simulink model "UnifiedPowerFlowController"  (R2024a)
settings: Solver=FixedStepDiscrete  StartTime=0.0  StopTime=0.8  FixedStep=Ts  RelTol=1e-3
PreLoadFcn:
  | Ts=1/512/60;
undefined symbols (not defined in the file or in its folder): DiscIntNeverNeededParam
libraries: spsabctodq0Lib x10, spsMeanVariableFrequencyLib x10, spsThreeLevelBridgeLib x8, spsVoltageMeasurementLib x8, spsZigzagPhaseShiftingTransformerLib x8, spsCurrentMeasurementLib x6, spsSecondOrderFilterLib x5, spsThreePhaseVIMeasurementLib x4, spsSeriesRLCBranchLib x4, spsDistributedParametersLineLib x3, spsPowerPositiveSequenceLib x3, spsThreePhaseSourceLib x2
(part 5 of 7)

== system UnifiedPowerFlowController/UPFC Controller/SE Control (SSSC)/Firing Pulses Generator/Bridge 1Y /Phase B ==
  note: <--Sigma-->
  note: |
      | |
      | |
  note: |
      | |
      | |
  note: Q4
  note: Q3
  note: Q2
  note: Q1
  note: ******************************************
  note: ********************************************
  note: ******************
  note: ******************
  note: 360
  note: 180
  note: 0
  note: I--------------------------------I-----------------------------I--
  note: Normal 180deg
      | Operation
  note: Normal 180deg
      | Operation
  note: Normal 180deg
      | Operation
  note: Pulses timing
      | ===========
  note: |
      | |
      | |
      | |
      | |
      | |
      | |
      | |
      | |
      | |
      | |
  note: |
      | |
      | |
      | |
      | |
      | |
      | |
      | |
      | |
      | |
      | |
  note: |
      | |
      | |
      | |
      | |
      | |
      | |
      | |
      | |
      | |
      | |
  note: Q1,Q2,Q3,Q4
  note: Q2,Q3
  note: Q4,Q1
  note: + Vdc -------------------------------
  note: - Vdc -------------------------------
  note: N -------
  note: |
      | |
      | |
      | |
      | |
      | |
      | |
      | |
      | |
      | |
      | |
  note: ---------- A
  note: --------[D-NN]---------
  note: --------[D_NP]---------
  note: |
      | |
      | [G4]
      | |
      | |
      | |
  note: |
      | |
      | [Q3]
      | |
      | |
  note: |
      | |
      | [Q2]
      | |
      | |
  note: |
      | |
      | |
      | [Q1]
      | |
      | |
  wt : Inport  PortDimensions=1
  sigma : Inport  Port=2  PortDimensions=1
  D_Alpha : Inport  Port=3  PortDimensions=1
  Constant1 : Constant  Value=[0 -pi]
  Constant2 : Constant  Value=2*pi
  Constant3 : Constant  Value=0
  Constant8 : Constant  Value=pi
  Constant9 : Constant  Value=pi
  Deg->Rad2 : Gain  Gain=0.5  SaturateOnIntegerOverflow=on  OutDataTypeStr=Inherit: Same as input  ParamDataTypeStr=Inherit: Same as input
  Deg->Rad3 : Gain  Gain=-1  SaturateOnIntegerOverflow=on  OutDataTypeStr=Inherit: Same as input  ParamDataTypeStr=Inherit: Same as input
  Gain3 : Gain  Gain=2  SaturateOnIntegerOverflow=on  OutDataTypeStr=Inherit: Same as input  ParamDataTypeStr=Inherit: Same as input
  Logical Operator : Logic
  Logical Operator2 : Logic  Operator=NOT
  Math Function : Math  Operator=mod  SignedPower=on
  Mux3 : Mux  Inputs=[2 2]
  Mux4 : Mux  Inputs=2
  Relational Operator : RelationalOperator
  Relational Operator1 : RelationalOperator  Operator=<
  Selector3 : Selector  InputPortWidth=4  IndexOptions=Index vector (dialog)  Indices=[4 1 2 3]  OutputSizes=1
  Sum{2,4..6} (4 alike) : Sum  InputSameDT=on  SaturateOnIntegerOverflow=on  OutDataTypeStr=Inherit: Same as first input
  Sum3 : Sum  Inputs=+-  InputSameDT=on  SaturateOnIntegerOverflow=on  OutDataTypeStr=Inherit: Same as first input
  Pulses : Outport  VectorParamsAs1DForOutWhenUnconnected=off
  wires:
  Constant2/1 -> Math Function/2
  Sum5/1 -> Sum2/1  "theta"
  wt/1 -> Sum5/1  "wt"
  D_Alpha/1 -> Mux4/1, Deg->Rad3/1
  Deg->Rad3/1 -> Mux4/2
  Mux4/1 -> Sum5/2
  Math Function/1 -> Relational Operator/1, Relational Operator1/1
  Gain3/1 -> Sum6/1
  Selector3/1 -> Pulses/1
  Mux3/1 -> Selector3/1
  Logical Operator2/1 -> Mux3/2
  Logical Operator/1 -> Mux3/1, Logical Operator2/1
  Sum4/1 -> Math Function/1
  Sum2/1 -> Sum4/2
  Sum6/1 -> Relational Operator1/2
  Constant8/1 -> Sum6/2
  Deg->Rad2/1 -> Gain3/1, Sum4/1  "Beta"
  Sum3/1 -> Deg->Rad2/1
  sigma/1 -> Sum3/2
  Constant9/1 -> Sum3/1
  Relational Operator1/1 -> Logical Operator/2
  Relational Operator/1 -> Logical Operator/1
  Constant3/1 -> Relational Operator/2
  Constant1/1 -> Sum2/2

== system UnifiedPowerFlowController/UPFC Controller/SE Control (SSSC)/Firing Pulses Generator/Bridge 1Y /Phase C ==
  note: |
      | |
      | |
      | [Q1]
      | |
      | |
  note: |
      | |
      | [Q2]
      | |
      | |
  note: |
      | |
      | [Q3]
      | |
      | |
  note: |
      | |
      | [G4]
      | |
      | |
      | |
  note: --------[D_NP]---------
  note: --------[D-NN]---------
  note: ---------- A
  note: |
      | |
      | |
      | |
      | |
      | |
      | |
      | |
      | |
      | |
      | |
  note: N -------
  note: - Vdc -------------------------------
  note: + Vdc -------------------------------
  note: Q4,Q1
  note: Q2,Q3
  note: Q1,Q2,Q3,Q4
  note: |
      | |
      | |
      | |
      | |
      | |
      | |
      | |
      | |
      | |
      | |
  note: |
      | |
      | |
      | |
      | |
      | |
      | |
      | |
      | |
      | |
      | |
  note: |
      | |
      | |
      | |
      | |
      | |
      | |
      | |
      | |
      | |
      | |
  note: Pulses timing
      | ===========
  note: Normal 180deg
      | Operation
  note: Normal 180deg
      | Operation
  note: Normal 180deg
      | Operation
  note: I--------------------------------I-----------------------------I--
  note: 0
  note: 180
  note: 360
  note: ******************
  note: ******************
  note: ********************************************
  note: ******************************************
  note: Q1
  note: Q2
  note: Q3
  note: Q4
  note: |
      | |
      | |
  note: |
      | |
      | |
  note: <--Sigma-->
  wt : Inport  PortDimensions=1
  sigma : Inport  Port=2  PortDimensions=1
  D_Alpha : Inport  Port=3  PortDimensions=1
  Constant1 : Constant  Value=[0 -pi]
  Constant2 : Constant  Value=2*pi
  Constant3 : Constant  Value=0
  Constant8 : Constant  Value=pi
  Constant9 : Constant  Value=pi
  Deg->Rad2 : Gain  Gain=0.5  SaturateOnIntegerOverflow=on  OutDataTypeStr=Inherit: Same as input  ParamDataTypeStr=Inherit: Same as input
  Deg->Rad3 : Gain  Gain=-1  SaturateOnIntegerOverflow=on  OutDataTypeStr=Inherit: Same as input  ParamDataTypeStr=Inherit: Same as input
  Gain3 : Gain  Gain=2  SaturateOnIntegerOverflow=on  OutDataTypeStr=Inherit: Same as input  ParamDataTypeStr=Inherit: Same as input
  Logical Operator : Logic
  Logical Operator2 : Logic  Operator=NOT
  Math Function : Math  Operator=mod  SignedPower=on
  Mux3 : Mux  Inputs=[2 2]
  Mux4 : Mux  Inputs=2
  Relational Operator : RelationalOperator
  Relational Operator1 : RelationalOperator  Operator=<
  Selector3 : Selector  InputPortWidth=4  IndexOptions=Index vector (dialog)  Indices=[4 1 2 3]  OutputSizes=1
  Sum{2,4..6} (4 alike) : Sum  InputSameDT=on  SaturateOnIntegerOverflow=on  OutDataTypeStr=Inherit: Same as first input
  Sum3 : Sum  Inputs=+-  InputSameDT=on  SaturateOnIntegerOverflow=on  OutDataTypeStr=Inherit: Same as first input
  Pulses : Outport  VectorParamsAs1DForOutWhenUnconnected=off
  wires:
  Constant1/1 -> Sum2/2
  Constant3/1 -> Relational Operator/2
  Relational Operator/1 -> Logical Operator/1
  Relational Operator1/1 -> Logical Operator/2
  Constant9/1 -> Sum3/1
  sigma/1 -> Sum3/2
  Sum3/1 -> Deg->Rad2/1
  Deg->Rad2/1 -> Sum4/1, Gain3/1  "Beta"
  Constant8/1 -> Sum6/2
  Sum6/1 -> Relational Operator1/2
  Sum2/1 -> Sum4/2
  Sum4/1 -> Math Function/1
  Logical Operator/1 -> Logical Operator2/1, Mux3/1
  Logical Operator2/1 -> Mux3/2
  Mux3/1 -> Selector3/1
  Selector3/1 -> Pulses/1
  Gain3/1 -> Sum6/1
  Math Function/1 -> Relational Operator1/1, Relational Operator/1
  Mux4/1 -> Sum5/2
  Deg->Rad3/1 -> Mux4/2
  D_Alpha/1 -> Deg->Rad3/1, Mux4/1
  wt/1 -> Sum5/1  "wt"
  Sum5/1 -> Sum2/1  "theta"
  Constant2/1 -> Math Function/2

== system UnifiedPowerFlowController/UPFC Controller/SE Control (SSSC)/Firing Pulses Generator/Bridge 2D/Phase A ==
  note: <--Sigma-->
  note: |
      | |
      | |
  note: |
      | |
      | |
  note: Q4
  note: Q3
  note: Q2
  note: Q1
  note: ******************************************
  note: ********************************************
  note: ******************
  note: ******************
  note: 360
  note: 180
  note: 0
  note: I--------------------------------I-----------------------------I--
  note: Normal 180deg
      | Operation
  note: Normal 180deg
      | Operation
  note: Normal 180deg
      | Operation
  note: Pulses timing
      | ===========
  note: |
      | |
      | |
      | |
      | |
      | |
      | |
      | |
      | |
      | |
      | |
  note: |
      | |
      | |
      | |
      | |
      | |
      | |
      | |
      | |
      | |
      | |
  note: |
      | |
      | |
      | |
      | |
      | |
      | |
      | |
      | |
      | |
      | |
  note: Q1,Q2,Q3,Q4
  note: Q2,Q3
  note: Q4,Q1
  note: + Vdc -------------------------------
  note: - Vdc -------------------------------
  note: N -------
  note: |
      | |
      | |
      | |
      | |
      | |
      | |
      | |
      | |
      | |
      | |
  note: ---------- A
  note: --------[D-NN]---------
  note: --------[D_NP]---------
  note: |
      | |
      | [G4]
      | |
      | |
      | |
  note: |
      | |
      | [Q3]
      | |
      | |
  note: |
      | |
      | [Q2]
      | |
      | |
  note: |
      | |
      | |
      | [Q1]
      | |
      | |
  wt : Inport  PortDimensions=1
  sigma : Inport  Port=2  PortDimensions=1
  D_Alpha : Inport  Port=3  PortDimensions=1
  Constant1 : Constant  Value=[0 -pi]
  Constant2 : Constant  Value=2*pi
  Constant3 : Constant  Value=0
  Constant8 : Constant  Value=pi
  Constant9 : Constant  Value=pi
  Deg->Rad2 : Gain  Gain=0.5  SaturateOnIntegerOverflow=on  OutDataTypeStr=Inherit: Same as input  ParamDataTypeStr=Inherit: Same as input
  Deg->Rad3 : Gain  Gain=-1  SaturateOnIntegerOverflow=on  OutDataTypeStr=Inherit: Same as input  ParamDataTypeStr=Inherit: Same as input
  Gain3 : Gain  Gain=2  SaturateOnIntegerOverflow=on  OutDataTypeStr=Inherit: Same as input  ParamDataTypeStr=Inherit: Same as input
  Logical Operator : Logic
  Logical Operator2 : Logic  Operator=NOT
  Math Function : Math  Operator=mod  SignedPower=on
  Mux3 : Mux  Inputs=[2 2]
  Mux4 : Mux  Inputs=2
  Relational Operator : RelationalOperator
  Relational Operator1 : RelationalOperator  Operator=<
  Selector3 : Selector  InputPortWidth=4  IndexOptions=Index vector (dialog)  Indices=[4 1 2 3]  OutputSizes=1
  Sum{2,4..6} (4 alike) : Sum  InputSameDT=on  SaturateOnIntegerOverflow=on  OutDataTypeStr=Inherit: Same as first input
  Sum3 : Sum  Inputs=+-  InputSameDT=on  SaturateOnIntegerOverflow=on  OutDataTypeStr=Inherit: Same as first input
  Pulses : Outport  VectorParamsAs1DForOutWhenUnconnected=off
  wires:
  Constant2/1 -> Math Function/2
  Sum5/1 -> Sum2/1  "theta"
  wt/1 -> Sum5/1  "wt"
  D_Alpha/1 -> Mux4/1, Deg->Rad3/1
  Deg->Rad3/1 -> Mux4/2
  Mux4/1 -> Sum5/2
  Math Function/1 -> Relational Operator/1, Relational Operator1/1
  Gain3/1 -> Sum6/1
  Selector3/1 -> Pulses/1
  Mux3/1 -> Selector3/1
  Logical Operator2/1 -> Mux3/2
  Logical Operator/1 -> Mux3/1, Logical Operator2/1
  Sum4/1 -> Math Function/1
  Sum2/1 -> Sum4/2
  Sum6/1 -> Relational Operator1/2
  Constant8/1 -> Sum6/2
  Deg->Rad2/1 -> Gain3/1, Sum4/1  "Beta"
  Sum3/1 -> Deg->Rad2/1
  sigma/1 -> Sum3/2
  Constant9/1 -> Sum3/1
  Relational Operator1/1 -> Logical Operator/2
  Relational Operator/1 -> Logical Operator/1
  Constant3/1 -> Relational Operator/2
  Constant1/1 -> Sum2/2

== system UnifiedPowerFlowController/UPFC Controller/SE Control (SSSC)/Firing Pulses Generator/Bridge 2D/Phase B ==
  note: |
      | |
      | |
      | [Q1]
      | |
      | |
  note: |
      | |
      | [Q2]
      | |
      | |
  note: |
      | |
      | [Q3]
      | |
      | |
  note: |
      | |
      | [G4]
      | |
      | |
      | |
  note: --------[D_NP]---------
  note: --------[D-NN]---------
  note: ---------- A
  note: |
      | |
      | |
      | |
      | |
      | |
      | |
      | |
      | |
      | |
      | |
  note: N -------
  note: - Vdc -------------------------------
  note: + Vdc -------------------------------
  note: Q4,Q1
  note: Q2,Q3
  note: Q1,Q2,Q3,Q4
  note: |
      | |
      | |
      | |
      | |
      | |
      | |
      | |
      | |
      | |
      | |
  note: |
      | |
      | |
      | |
      | |
      | |
      | |
      | |
      | |
      | |
      | |
  note: |
      | |
      | |
      | |
      | |
      | |
      | |
      | |
      | |
      | |
      | |
  note: Pulses timing
      | ===========
  note: Normal 180deg
      | Operation
  note: Normal 180deg
      | Operation
  note: Normal 180deg
      | Operation
  note: I--------------------------------I-----------------------------I--
  note: 0
  note: 180
  note: 360
  note: ******************
  note: ******************
  note: ********************************************
  note: ******************************************
  note: Q1
  note: Q2
  note: Q3
  note: Q4
  note: |
      | |
      | |
  note: |
      | |
      | |
  note: <--Sigma-->
  wt : Inport  PortDimensions=1
  sigma : Inport  Port=2  PortDimensions=1
  D_Alpha : Inport  Port=3  PortDimensions=1
  Constant1 : Constant  Value=[0 -pi]
  Constant2 : Constant  Value=2*pi
  Constant3 : Constant  Value=0
  Constant8 : Constant  Value=pi
  Constant9 : Constant  Value=pi
  Deg->Rad2 : Gain  Gain=0.5  SaturateOnIntegerOverflow=on  OutDataTypeStr=Inherit: Same as input  ParamDataTypeStr=Inherit: Same as input
  Deg->Rad3 : Gain  Gain=-1  SaturateOnIntegerOverflow=on  OutDataTypeStr=Inherit: Same as input  ParamDataTypeStr=Inherit: Same as input
  Gain3 : Gain  Gain=2  SaturateOnIntegerOverflow=on  OutDataTypeStr=Inherit: Same as input  ParamDataTypeStr=Inherit: Same as input
  Logical Operator : Logic
  Logical Operator2 : Logic  Operator=NOT
  Math Function : Math  Operator=mod  SignedPower=on
  Mux3 : Mux  Inputs=[2 2]
  Mux4 : Mux  Inputs=2
  Relational Operator : RelationalOperator
  Relational Operator1 : RelationalOperator  Operator=<
  Selector3 : Selector  InputPortWidth=4  IndexOptions=Index vector (dialog)  Indices=[4 1 2 3]  OutputSizes=1
  Sum{2,4..6} (4 alike) : Sum  InputSameDT=on  SaturateOnIntegerOverflow=on  OutDataTypeStr=Inherit: Same as first input
  Sum3 : Sum  Inputs=+-  InputSameDT=on  SaturateOnIntegerOverflow=on  OutDataTypeStr=Inherit: Same as first input
  Pulses : Outport  VectorParamsAs1DForOutWhenUnconnected=off
  wires:
  Constant1/1 -> Sum2/2
  Constant3/1 -> Relational Operator/2
  Relational Operator/1 -> Logical Operator/1
  Relational Operator1/1 -> Logical Operator/2
  Constant9/1 -> Sum3/1
  sigma/1 -> Sum3/2
  Sum3/1 -> Deg->Rad2/1
  Deg->Rad2/1 -> Sum4/1, Gain3/1  "Beta"
  Constant8/1 -> Sum6/2
  Sum6/1 -> Relational Operator1/2
  Sum2/1 -> Sum4/2
  Sum4/1 -> Math Function/1
  Logical Operator/1 -> Logical Operator2/1, Mux3/1
  Logical Operator2/1 -> Mux3/2
  Mux3/1 -> Selector3/1
  Selector3/1 -> Pulses/1
  Gain3/1 -> Sum6/1
  Math Function/1 -> Relational Operator1/1, Relational Operator/1
  Mux4/1 -> Sum5/2
  Deg->Rad3/1 -> Mux4/2
  D_Alpha/1 -> Deg->Rad3/1, Mux4/1
  wt/1 -> Sum5/1  "wt"
  Sum5/1 -> Sum2/1  "theta"
  Constant2/1 -> Math Function/2

== system UnifiedPowerFlowController/UPFC Controller/SE Control (SSSC)/Firing Pulses Generator/Bridge 2D/Phase C ==
  note: <--Sigma-->
  note: |
      | |
      | |
  note: |
      | |
      | |
  note: Q4
  note: Q3
  note: Q2
  note: Q1
  note: ******************************************
  note: ********************************************
  note: ******************
  note: ******************
  note: 360
  note: 180
  note: 0
  note: I--------------------------------I-----------------------------I--
  note: Normal 180deg
      | Operation
  note: Normal 180deg
      | Operation
  note: Normal 180deg
      | Operation
  note: Pulses timing
      | ===========
  note: |
      | |
      | |
      | |
      | |
      | |
      | |
      | |
      | |
      | |
      | |
  note: |
      | |
      | |
      | |
      | |
      | |
      | |
      | |
      | |
      | |
      | |
  note: |
      | |
      | |
      | |
      | |
      | |
      | |
      | |
      | |
      | |
      | |
  note: Q1,Q2,Q3,Q4
  note: Q2,Q3
  note: Q4,Q1
  note: + Vdc -------------------------------
  note: - Vdc -------------------------------
  note: N -------
  note: |
      | |
      | |
      | |
      | |
      | |
      | |
      | |
      | |
      | |
      | |
  note: ---------- A
  note: --------[D-NN]---------
  note: --------[D_NP]---------
  note: |
      | |
      | [G4]
      | |
      | |
      | |
  note: |
      | |
      | [Q3]
      | |
      | |
  note: |
      | |
      | [Q2]
      | |
      | |
  note: |
      | |
      | |
      | [Q1]
      | |
      | |
  wt : Inport  PortDimensions=1
  sigma : Inport  Port=2  PortDimensions=1
  D_Alpha : Inport  Port=3  PortDimensions=1
  Constant1 : Constant  Value=[0 -pi]
  Constant2 : Constant  Value=2*pi
  Constant3 : Constant  Value=0
  Constant8 : Constant  Value=pi
  Constant9 : Constant  Value=pi
  Deg->Rad2 : Gain  Gain=0.5  SaturateOnIntegerOverflow=on  OutDataTypeStr=Inherit: Same as input  ParamDataTypeStr=Inherit: Same as input
  Deg->Rad3 : Gain  Gain=-1  SaturateOnIntegerOverflow=on  OutDataTypeStr=Inherit: Same as input  ParamDataTypeStr=Inherit: Same as input
  Gain3 : Gain  Gain=2  SaturateOnIntegerOverflow=on  OutDataTypeStr=Inherit: Same as input  ParamDataTypeStr=Inherit: Same as input
  Logical Operator : Logic
  Logical Operator2 : Logic  Operator=NOT
  Math Function : Math  Operator=mod  SignedPower=on
  Mux3 : Mux  Inputs=[2 2]
  Mux4 : Mux  Inputs=2
  Relational Operator : RelationalOperator
  Relational Operator1 : RelationalOperator  Operator=<
  Selector3 : Selector  InputPortWidth=4  IndexOptions=Index vector (dialog)  Indices=[4 1 2 3]  OutputSizes=1
  Sum{2,4..6} (4 alike) : Sum  InputSameDT=on  SaturateOnIntegerOverflow=on  OutDataTypeStr=Inherit: Same as first input
  Sum3 : Sum  Inputs=+-  InputSameDT=on  SaturateOnIntegerOverflow=on  OutDataTypeStr=Inherit: Same as first input
  Pulses : Outport  VectorParamsAs1DForOutWhenUnconnected=off
  wires:
  Constant2/1 -> Math Function/2
  Sum5/1 -> Sum2/1  "theta"
  wt/1 -> Sum5/1  "wt"
  D_Alpha/1 -> Mux4/1, Deg->Rad3/1
  Deg->Rad3/1 -> Mux4/2
  Mux4/1 -> Sum5/2
  Math Function/1 -> Relational Operator/1, Relational Operator1/1
  Gain3/1 -> Sum6/1
  Selector3/1 -> Pulses/1
  Mux3/1 -> Selector3/1
  Logical Operator2/1 -> Mux3/2
  Logical Operator/1 -> Mux3/1, Logical Operator2/1
  Sum4/1 -> Math Function/1
  Sum2/1 -> Sum4/2
  Sum6/1 -> Relational Operator1/2
  Constant8/1 -> Sum6/2
  Deg->Rad2/1 -> Gain3/1, Sum4/1  "Beta"
  Sum3/1 -> Deg->Rad2/1
  sigma/1 -> Sum3/2
  Constant9/1 -> Sum3/1
  Relational Operator1/1 -> Logical Operator/2
  Relational Operator/1 -> Logical Operator/1
  Constant3/1 -> Relational Operator/2
  Constant1/1 -> Sum2/2

== system UnifiedPowerFlowController/UPFC Controller/SE Control (SSSC)/Firing Pulses Generator/Bridge 2Y/Phase A ==
  note: |
      | |
      | |
      | [Q1]
      | |
      | |
  note: |
      | |
      | [Q2]
      | |
      | |
  note: |
      | |
      | [Q3]
      | |
      | |
  note: |
      | |
      | [G4]
      | |
      | |
      | |
  note: --------[D_NP]---------
  note: --------[D-NN]---------
  note: ---------- A
  note: |
      | |
      | |
      | |
      | |
      | |
      | |
      | |
      | |
      | |
      | |
  note: N -------
  note: - Vdc -------------------------------
  note: + Vdc -------------------------------
  note: Q4,Q1
  note: Q2,Q3
  note: Q1,Q2,Q3,Q4
  note: |
      | |
      | |
      | |
      | |
      | |
      | |
      | |
      | |
      | |
      | |
  note: |
      | |
      | |
      | |
      | |
      | |
      | |
      | |
      | |
      | |
      | |
  note: |
      | |
      | |
      | |
      | |
      | |
      | |
      | |
      | |
      | |
      | |
  note: Pulses timing
      | ===========
  note: Normal 180deg
      | Operation
  note: Normal 180deg
      | Operation
  note: Normal 180deg
      | Operation
  note: I--------------------------------I-----------------------------I--
  note: 0
  note: 180
  note: 360
  note: ******************
  note: ******************
  note: ********************************************
  note: ******************************************
  note: Q1
  note: Q2
  note: Q3
  note: Q4
  note: |
      | |
      | |
  note: |
      | |
      | |
  note: <--Sigma-->
  wt : Inport  PortDimensions=1
  sigma : Inport  Port=2  PortDimensions=1
  D_Alpha : Inport  Port=3  PortDimensions=1
  Constant1 : Constant  Value=[0 -pi]
  Constant2 : Constant  Value=2*pi
  Constant3 : Constant  Value=0
  Constant8 : Constant  Value=pi
  Constant9 : Constant  Value=pi
  Deg->Rad2 : Gain  Gain=0.5  SaturateOnIntegerOverflow=on  OutDataTypeStr=Inherit: Same as input  ParamDataTypeStr=Inherit: Same as input
  Deg->Rad3 : Gain  Gain=-1  SaturateOnIntegerOverflow=on  OutDataTypeStr=Inherit: Same as input  ParamDataTypeStr=Inherit: Same as input
  Gain3 : Gain  Gain=2  SaturateOnIntegerOverflow=on  OutDataTypeStr=Inherit: Same as input  ParamDataTypeStr=Inherit: Same as input
  Logical Operator : Logic
  Logical Operator2 : Logic  Operator=NOT
  Math Function : Math  Operator=mod  SignedPower=on
  Mux3 : Mux  Inputs=[2 2]
  Mux4 : Mux  Inputs=2
  Relational Operator : RelationalOperator
  Relational Operator1 : RelationalOperator  Operator=<
  Selector3 : Selector  InputPortWidth=4  IndexOptions=Index vector (dialog)  Indices=[4 1 2 3]  OutputSizes=1
  Sum{2,4..6} (4 alike) : Sum  InputSameDT=on  SaturateOnIntegerOverflow=on  OutDataTypeStr=Inherit: Same as first input
  Sum3 : Sum  Inputs=+-  InputSameDT=on  SaturateOnIntegerOverflow=on  OutDataTypeStr=Inherit: Same as first input
  Pulses : Outport  VectorParamsAs1DForOutWhenUnconnected=off
  wires:
  Constant1/1 -> Sum2/2
  Constant3/1 -> Relational Operator/2
  Relational Operator/1 -> Logical Operator/1
  Relational Operator1/1 -> Logical Operator/2
  Constant9/1 -> Sum3/1
  sigma/1 -> Sum3/2
  Sum3/1 -> Deg->Rad2/1
  Deg->Rad2/1 -> Sum4/1, Gain3/1  "Beta"
  Constant8/1 -> Sum6/2
  Sum6/1 -> Relational Operator1/2
  Sum2/1 -> Sum4/2
  Sum4/1 -> Math Function/1
  Logical Operator/1 -> Logical Operator2/1, Mux3/1
  Logical Operator2/1 -> Mux3/2
  Mux3/1 -> Selector3/1
  Selector3/1 -> Pulses/1
  Gain3/1 -> Sum6/1
  Math Function/1 -> Relational Operator1/1, Relational Operator/1
  Mux4/1 -> Sum5/2
  Deg->Rad3/1 -> Mux4/2
  D_Alpha/1 -> Deg->Rad3/1, Mux4/1
  wt/1 -> Sum5/1  "wt"
  Sum5/1 -> Sum2/1  "theta"
  Constant2/1 -> Math Function/2

== system UnifiedPowerFlowController/UPFC Controller/SE Control (SSSC)/Firing Pulses Generator/Bridge 2Y/Phase B ==
  note: <--Sigma-->
  note: |
      | |
      | |
  note: |
      | |
      | |
  note: Q4
  note: Q3
  note: Q2
  note: Q1
  note: ******************************************
  note: ********************************************
  note: ******************
  note: ******************
  note: 360
  note: 180
  note: 0
  note: I--------------------------------I-----------------------------I--
  note: Normal 180deg
      | Operation
  note: Normal 180deg
      | Operation
  note: Normal 180deg
      | Operation
  note: Pulses timing
      | ===========
  note: |
      | |
      | |
      | |
      | |
      | |
      | |
      | |
      | |
      | |
      | |
  note: |
      | |
      | |
      | |
      | |
      | |
      | |
      | |
      | |
      | |
      | |
  note: |
      | |
      | |
      | |
      | |
      | |
      | |
      | |
      | |
      | |
      | |
  note: Q1,Q2,Q3,Q4
  note: Q2,Q3
  note: Q4,Q1
  note: + Vdc -------------------------------
  note: - Vdc -------------------------------
  note: N -------
  note: |
      | |
      | |
      | |
      | |
      | |
      | |
      | |
      | |
      | |
      | |
  note: ---------- A
  note: --------[D-NN]---------
  note: --------[D_NP]---------
  note: |
      | |
      | [G4]
      | |
      | |
      | |
  note: |
      | |
      | [Q3]
      | |
      | |
  note: |
      | |
      | [Q2]
      | |
      | |
  note: |
      | |
      | |
      | [Q1]
      | |
      | |
  wt : Inport  PortDimensions=1
  sigma : Inport  Port=2  PortDimensions=1
  D_Alpha : Inport  Port=3  PortDimensions=1
  Constant1 : Constant  Value=[0 -pi]
  Constant2 : Constant  Value=2*pi
  Constant3 : Constant  Value=0
  Constant8 : Constant  Value=pi
  Constant9 : Constant  Value=pi
  Deg->Rad2 : Gain  Gain=0.5  SaturateOnIntegerOverflow=on  OutDataTypeStr=Inherit: Same as input  ParamDataTypeStr=Inherit: Same as input
  Deg->Rad3 : Gain  Gain=-1  SaturateOnIntegerOverflow=on  OutDataTypeStr=Inherit: Same as input  ParamDataTypeStr=Inherit: Same as input
  Gain3 : Gain  Gain=2  SaturateOnIntegerOverflow=on  OutDataTypeStr=Inherit: Same as input  ParamDataTypeStr=Inherit: Same as input
  Logical Operator : Logic
  Logical Operator2 : Logic  Operator=NOT
  Math Function : Math  Operator=mod  SignedPower=on
  Mux3 : Mux  Inputs=[2 2]
  Mux4 : Mux  Inputs=2
  Relational Operator : RelationalOperator
  Relational Operator1 : RelationalOperator  Operator=<
  Selector3 : Selector  InputPortWidth=4  IndexOptions=Index vector (dialog)  Indices=[4 1 2 3]  OutputSizes=1
  Sum{2,4..6} (4 alike) : Sum  InputSameDT=on  SaturateOnIntegerOverflow=on  OutDataTypeStr=Inherit: Same as first input
  Sum3 : Sum  Inputs=+-  InputSameDT=on  SaturateOnIntegerOverflow=on  OutDataTypeStr=Inherit: Same as first input
  Pulses : Outport  VectorParamsAs1DForOutWhenUnconnected=off
  wires:
  Constant2/1 -> Math Function/2
  Sum5/1 -> Sum2/1  "theta"
  wt/1 -> Sum5/1  "wt"
  D_Alpha/1 -> Mux4/1, Deg->Rad3/1
  Deg->Rad3/1 -> Mux4/2
  Mux4/1 -> Sum5/2
  Math Function/1 -> Relational Operator/1, Relational Operator1/1
  Gain3/1 -> Sum6/1
  Selector3/1 -> Pulses/1
  Mux3/1 -> Selector3/1
  Logical Operator2/1 -> Mux3/2
  Logical Operator/1 -> Mux3/1, Logical Operator2/1
  Sum4/1 -> Math Function/1
  Sum2/1 -> Sum4/2
  Sum6/1 -> Relational Operator1/2
  Constant8/1 -> Sum6/2
  Deg->Rad2/1 -> Gain3/1, Sum4/1  "Beta"
  Sum3/1 -> Deg->Rad2/1
  sigma/1 -> Sum3/2
  Constant9/1 -> Sum3/1
  Relational Operator1/1 -> Logical Operator/2
  Relational Operator/1 -> Logical Operator/1
  Constant3/1 -> Relational Operator/2
  Constant1/1 -> Sum2/2

== system UnifiedPowerFlowController/UPFC Controller/SE Control (SSSC)/Firing Pulses Generator/Bridge 2Y/Phase C ==
  note: |
      | |
      | |
      | [Q1]
      | |
      | |
  note: |
      | |
      | [Q2]
      | |
      | |
  note: |
      | |
      | [Q3]
      | |
      | |
  note: |
      | |
      | [G4]
      | |
      | |
      | |
  note: --------[D_NP]---------
  note: --------[D-NN]---------
  note: ---------- A
  note: |
      | |
      | |
      | |
      | |
      | |
      | |
      | |
      | |
      | |
      | |
  note: N -------
  note: - Vdc -------------------------------
  note: + Vdc -------------------------------
  note: Q4,Q1
  note: Q2,Q3
  note: Q1,Q2,Q3,Q4
  note: |
      | |
      | |
      | |
      | |
      | |
      | |
      | |
      | |
      | |
      | |
  note: |
      | |
      | |
      | |
      | |
      | |
      | |
      | |
      | |
      | |
      | |
  note: |
      | |
      | |
      | |
      | |
      | |
      | |
      | |
      | |
      | |
      | |
  note: Pulses timing
      | ===========
  note: Normal 180deg
      | Operation
  note: Normal 180deg
      | Operation
  note: Normal 180deg
      | Operation
  note: I--------------------------------I-----------------------------I--
  note: 0
  note: 180
  note: 360
  note: ******************
  note: ******************
  note: ********************************************
  note: ******************************************
  note: Q1
  note: Q2
  note: Q3
  note: Q4
  note: |
      | |
      | |
  note: |
      | |
      | |
  note: <--Sigma-->
  wt : Inport  PortDimensions=1
  sigma : Inport  Port=2  PortDimensions=1
  D_Alpha : Inport  Port=3  PortDimensions=1
  Constant1 : Constant  Value=[0 -pi]
  Constant2 : Constant  Value=2*pi
  Constant3 : Constant  Value=0
  Constant8 : Constant  Value=pi
  Constant9 : Constant  Value=pi
  Deg->Rad2 : Gain  Gain=0.5  SaturateOnIntegerOverflow=on  OutDataTypeStr=Inherit: Same as input  ParamDataTypeStr=Inherit: Same as input
  Deg->Rad3 : Gain  Gain=-1  SaturateOnIntegerOverflow=on  OutDataTypeStr=Inherit: Same as input  ParamDataTypeStr=Inherit: Same as input
  Gain3 : Gain  Gain=2  SaturateOnIntegerOverflow=on  OutDataTypeStr=Inherit: Same as input  ParamDataTypeStr=Inherit: Same as input
  Logical Operator : Logic
  Logical Operator2 : Logic  Operator=NOT
  Math Function : Math  Operator=mod  SignedPower=on
  Mux3 : Mux  Inputs=[2 2]
  Mux4 : Mux  Inputs=2
  Relational Operator : RelationalOperator
  Relational Operator1 : RelationalOperator  Operator=<
  Selector3 : Selector  InputPortWidth=4  IndexOptions=Index vector (dialog)  Indices=[4 1 2 3]  OutputSizes=1
  Sum{2,4..6} (4 alike) : Sum  InputSameDT=on  SaturateOnIntegerOverflow=on  OutDataTypeStr=Inherit: Same as first input
  Sum3 : Sum  Inputs=+-  InputSameDT=on  SaturateOnIntegerOverflow=on  OutDataTypeStr=Inherit: Same as first input
  Pulses : Outport  VectorParamsAs1DForOutWhenUnconnected=off
  wires:
  Constant1/1 -> Sum2/2
  Constant3/1 -> Relational Operator/2
  Relational Operator/1 -> Logical Operator/1
  Relational Operator1/1 -> Logical Operator/2
  Constant9/1 -> Sum3/1
  sigma/1 -> Sum3/2
  Sum3/1 -> Deg->Rad2/1
  Deg->Rad2/1 -> Sum4/1, Gain3/1  "Beta"
  Constant8/1 -> Sum6/2
  Sum6/1 -> Relational Operator1/2
  Sum2/1 -> Sum4/2
  Sum4/1 -> Math Function/1
  Logical Operator/1 -> Logical Operator2/1, Mux3/1
  Logical Operator2/1 -> Mux3/2
  Mux3/1 -> Selector3/1
  Selector3/1 -> Pulses/1
  Gain3/1 -> Sum6/1
  Math Function/1 -> Relational Operator1/1, Relational Operator/1
  Mux4/1 -> Sum5/2
  Deg->Rad3/1 -> Mux4/2
  D_Alpha/1 -> Deg->Rad3/1, Mux4/1
  wt/1 -> Sum5/1  "wt"
  Sum5/1 -> Sum2/1  "theta"
  Constant2/1 -> Math Function/2

== system UnifiedPowerFlowController/UPFC Controller/SE Control (UPFC)/Firing Pulses Generator/Bridge 1D/Phase A ==
  note: <--Sigma-->
  note: |
      | |
      | |
  note: |
      | |
      | |
  note: Q4
  note: Q3
  note: Q2
  note: Q1
  note: ******************************************
  note: ********************************************
  note: ******************
  note: ******************
  note: 360
  note: 180
  note: 0
  note: I--------------------------------I-----------------------------I--
  note: Normal 180deg
      | Operation
  note: Normal 180deg
      | Operation
  note: Normal 180deg
      | Operation
  note: Pulses timing
      | ===========
  note: |
      | |
      | |
      | |
      | |
      | |
      | |
      | |
      | |
      | |
      | |
  note: |
      | |
      | |
      | |
      | |
      | |
      | |
      | |
      | |
      | |
      | |
  note: |
      | |
      | |
      | |
      | |
      | |
      | |
      | |
      | |
      | |
      | |
  note: Q1,Q2,Q3,Q4
  note: Q2,Q3
  note: Q4,Q1
  note: + Vdc -------------------------------
  note: - Vdc -------------------------------
  note: N -------
  note: |
      | |
      | |
      | |
      | |
      | |
      | |
      | |
      | |
      | |
      | |
  note: ---------- A
  note: --------[D-NN]---------
  note: --------[D_NP]---------
  note: |
      | |
      | [G4]
      | |
      | |
      | |
  note: |
      | |
      | [Q3]
      | |
      | |
  note: |
      | |
      | [Q2]
      | |
      | |
  note: |
      | |
      | |
      | [Q1]
      | |
      | |
  wt : Inport  PortDimensions=1
  sigma : Inport  Port=2  PortDimensions=1
  D_Alpha : Inport  Port=3  PortDimensions=1
  Constant1 : Constant  Value=[0 -pi]
  Constant2 : Constant  Value=2*pi
  Constant3 : Constant  Value=0
  Constant8 : Constant  Value=pi
  Constant9 : Constant  Value=pi
  Deg->Rad2 : Gain  Gain=0.5  SaturateOnIntegerOverflow=on  OutDataTypeStr=Inherit: Same as input  ParamDataTypeStr=Inherit: Same as input
  Deg->Rad3 : Gain  Gain=-1  SaturateOnIntegerOverflow=on  OutDataTypeStr=Inherit: Same as input  ParamDataTypeStr=Inherit: Same as input
  Gain3 : Gain  Gain=2  SaturateOnIntegerOverflow=on  OutDataTypeStr=Inherit: Same as input  ParamDataTypeStr=Inherit: Same as input
  Logical Operator : Logic
  Logical Operator2 : Logic  Operator=NOT
  Math Function : Math  Operator=mod  SignedPower=on
  Mux3 : Mux  Inputs=[2 2]
  Mux4 : Mux  Inputs=2
  Relational Operator : RelationalOperator
  Relational Operator1 : RelationalOperator  Operator=<
  Selector3 : Selector  InputPortWidth=4  IndexOptions=Index vector (dialog)  Indices=[4 1 2 3]  OutputSizes=1
  Sum{2,4..6} (4 alike) : Sum  InputSameDT=on  SaturateOnIntegerOverflow=on  OutDataTypeStr=Inherit: Same as first input
  Sum3 : Sum  Inputs=+-  InputSameDT=on  SaturateOnIntegerOverflow=on  OutDataTypeStr=Inherit: Same as first input
  Pulses : Outport  VectorParamsAs1DForOutWhenUnconnected=off
  wires:
  Constant2/1 -> Math Function/2
  Sum5/1 -> Sum2/1  "theta"
  wt/1 -> Sum5/1  "wt"
  D_Alpha/1 -> Mux4/1, Deg->Rad3/1
  Deg->Rad3/1 -> Mux4/2
  Mux4/1 -> Sum5/2
  Math Function/1 -> Relational Operator/1, Relational Operator1/1
  Gain3/1 -> Sum6/1
  Selector3/1 -> Pulses/1
  Mux3/1 -> Selector3/1
  Logical Operator2/1 -> Mux3/2
  Logical Operator/1 -> Mux3/1, Logical Operator2/1
  Sum4/1 -> Math Function/1
  Sum2/1 -> Sum4/2
  Sum6/1 -> Relational Operator1/2
  Constant8/1 -> Sum6/2
  Deg->Rad2/1 -> Gain3/1, Sum4/1  "Beta"
  Sum3/1 -> Deg->Rad2/1
  sigma/1 -> Sum3/2
  Constant9/1 -> Sum3/1
  Relational Operator1/1 -> Logical Operator/2
  Relational Operator/1 -> Logical Operator/1
  Constant3/1 -> Relational Operator/2
  Constant1/1 -> Sum2/2

== system UnifiedPowerFlowController/UPFC Controller/SE Control (UPFC)/Firing Pulses Generator/Bridge 1D/Phase B ==
  note: |
      | |
      | |
      | [Q1]
      | |
      | |
  note: |
      | |
      | [Q2]
      | |
      | |
  note: |
      | |
      | [Q3]
      | |
      | |
  note: |
      | |
      | [G4]
      | |
      | |
      | |
  note: --------[D_NP]---------
  note: --------[D-NN]---------
  note: ---------- A
  note: |
      | |
      | |
      | |
      | |
      | |
      | |
      | |
      | |
      | |
      | |
  note: N -------
  note: - Vdc -------------------------------
  note: + Vdc -------------------------------
  note: Q4,Q1
  note: Q2,Q3
  note: Q1,Q2,Q3,Q4
  note: |
      | |
      | |
      | |
      | |
      | |
      | |
      | |
      | |
      | |
      | |
  note: |
      | |
      | |
      | |
      | |
      | |
      | |
      | |
      | |
      | |
      | |
  note: |
      | |
      | |
      | |
      | |
      | |
      | |
      | |
      | |
      | |
      | |
  note: Pulses timing
      | ===========
  note: Normal 180deg
      | Operation
  note: Normal 180deg
      | Operation
  note: Normal 180deg
      | Operation
  note: I--------------------------------I-----------------------------I--
  note: 0
  note: 180
  note: 360
  note: ******************
  note: ******************
  note: ********************************************
  note: ******************************************
  note: Q1
  note: Q2
  note: Q3
  note: Q4
  note: |
      | |
      | |
  note: |
      | |
      | |
  note: <--Sigma-->
  wt : Inport  PortDimensions=1
  sigma : Inport  Port=2  PortDimensions=1
  D_Alpha : Inport  Port=3  PortDimensions=1
  Constant1 : Constant  Value=[0 -pi]
  Constant2 : Constant  Value=2*pi
  Constant3 : Constant  Value=0
  Constant8 : Constant  Value=pi
  Constant9 : Constant  Value=pi
  Deg->Rad2 : Gain  Gain=0.5  SaturateOnIntegerOverflow=on  OutDataTypeStr=Inherit: Same as input  ParamDataTypeStr=Inherit: Same as input
  Deg->Rad3 : Gain  Gain=-1  SaturateOnIntegerOverflow=on  OutDataTypeStr=Inherit: Same as input  ParamDataTypeStr=Inherit: Same as input
  Gain3 : Gain  Gain=2  SaturateOnIntegerOverflow=on  OutDataTypeStr=Inherit: Same as input  ParamDataTypeStr=Inherit: Same as input
  Logical Operator : Logic
  Logical Operator2 : Logic  Operator=NOT
  Math Function : Math  Operator=mod  SignedPower=on
  Mux3 : Mux  Inputs=[2 2]
  Mux4 : Mux  Inputs=2
  Relational Operator : RelationalOperator
  Relational Operator1 : RelationalOperator  Operator=<
  Selector3 : Selector  InputPortWidth=4  IndexOptions=Index vector (dialog)  Indices=[4 1 2 3]  OutputSizes=1
  Sum{2,4..6} (4 alike) : Sum  InputSameDT=on  SaturateOnIntegerOverflow=on  OutDataTypeStr=Inherit: Same as first input
  Sum3 : Sum  Inputs=+-  InputSameDT=on  SaturateOnIntegerOverflow=on  OutDataTypeStr=Inherit: Same as first input
  Pulses : Outport  VectorParamsAs1DForOutWhenUnconnected=off
  wires:
  Constant1/1 -> Sum2/2
  Constant3/1 -> Relational Operator/2
  Relational Operator/1 -> Logical Operator/1
  Relational Operator1/1 -> Logical Operator/2
  Constant9/1 -> Sum3/1
  sigma/1 -> Sum3/2
  Sum3/1 -> Deg->Rad2/1
  Deg->Rad2/1 -> Sum4/1, Gain3/1  "Beta"
  Constant8/1 -> Sum6/2
  Sum6/1 -> Relational Operator1/2
  Sum2/1 -> Sum4/2
  Sum4/1 -> Math Function/1
  Logical Operator/1 -> Logical Operator2/1, Mux3/1
  Logical Operator2/1 -> Mux3/2
  Mux3/1 -> Selector3/1
  Selector3/1 -> Pulses/1
  Gain3/1 -> Sum6/1
  Math Function/1 -> Relational Operator1/1, Relational Operator/1
  Mux4/1 -> Sum5/2
  Deg->Rad3/1 -> Mux4/2
  D_Alpha/1 -> Deg->Rad3/1, Mux4/1
  wt/1 -> Sum5/1  "wt"
  Sum5/1 -> Sum2/1  "theta"
  Constant2/1 -> Math Function/2

== system UnifiedPowerFlowController/UPFC Controller/SE Control (UPFC)/Firing Pulses Generator/Bridge 1D/Phase C ==
  note: <--Sigma-->
  note: |
      | |
      | |
  note: |
      | |
      | |
  note: Q4
  note: Q3
  note: Q2
  note: Q1
  note: ******************************************
  note: ********************************************
  note: ******************
  note: ******************
  note: 360
  note: 180
  note: 0
  note: I--------------------------------I-----------------------------I--
  note: Normal 180deg
      | Operation
  note: Normal 180deg
      | Operation
  note: Normal 180deg
      | Operation
  note: Pulses timing
      | ===========
  note: |
      | |
      | |
      | |
      | |
      | |
      | |
      | |
      | |
      | |
      | |
  note: |
      | |
      | |
      | |
      | |
      | |
      | |
      | |
      | |
      | |
      | |
  note: |
      | |
      | |
      | |
      | |
      | |
      | |
      | |
      | |
      | |
      | |
  note: Q1,Q2,Q3,Q4
  note: Q2,Q3
  note: Q4,Q1
  note: + Vdc -------------------------------
  note: - Vdc -------------------------------
  note: N -------
  note: |
      | |
      | |
      | |
      | |
      | |
      | |
      | |
      | |
      | |
      | |
  note: ---------- A
  note: --------[D-NN]---------
  note: --------[D_NP]---------
  note: |
      | |
      | [G4]
      | |
      | |
      | |
  note: |
      | |
      | [Q3]
      | |
      | |
  note: |
      | |
      | [Q2]
      | |
      | |
  note: |
      | |
      | |
      | [Q1]
      | |
      | |
  wt : Inport  PortDimensions=1
  sigma : Inport  Port=2  PortDimensions=1
  D_Alpha : Inport  Port=3  PortDimensions=1
  Constant1 : Constant  Value=[0 -pi]
  Constant2 : Constant  Value=2*pi
  Constant3 : Constant  Value=0
  Constant8 : Constant  Value=pi
  Constant9 : Constant  Value=pi
  Deg->Rad2 : Gain  Gain=0.5  SaturateOnIntegerOverflow=on  OutDataTypeStr=Inherit: Same as input  ParamDataTypeStr=Inherit: Same as input
  Deg->Rad3 : Gain  Gain=-1  SaturateOnIntegerOverflow=on  OutDataTypeStr=Inherit: Same as input  ParamDataTypeStr=Inherit: Same as input
  Gain3 : Gain  Gain=2  SaturateOnIntegerOverflow=on  OutDataTypeStr=Inherit: Same as input  ParamDataTypeStr=Inherit: Same as input
  Logical Operator : Logic
  Logical Operator2 : Logic  Operator=NOT
  Math Function : Math  Operator=mod  SignedPower=on
  Mux3 : Mux  Inputs=[2 2]
  Mux4 : Mux  Inputs=2
  Relational Operator : RelationalOperator
  Relational Operator1 : RelationalOperator  Operator=<
  Selector3 : Selector  InputPortWidth=4  IndexOptions=Index vector (dialog)  Indices=[4 1 2 3]  OutputSizes=1
  Sum{2,4..6} (4 alike) : Sum  InputSameDT=on  SaturateOnIntegerOverflow=on  OutDataTypeStr=Inherit: Same as first input
  Sum3 : Sum  Inputs=+-  InputSameDT=on  SaturateOnIntegerOverflow=on  OutDataTypeStr=Inherit: Same as first input
  Pulses : Outport  VectorParamsAs1DForOutWhenUnconnected=off
  wires:
  Constant2/1 -> Math Function/2
  Sum5/1 -> Sum2/1  "theta"
  wt/1 -> Sum5/1  "wt"
  D_Alpha/1 -> Mux4/1, Deg->Rad3/1
  Deg->Rad3/1 -> Mux4/2
  Mux4/1 -> Sum5/2
  Math Function/1 -> Relational Operator/1, Relational Operator1/1
  Gain3/1 -> Sum6/1
  Selector3/1 -> Pulses/1
  Mux3/1 -> Selector3/1
  Logical Operator2/1 -> Mux3/2
  Logical Operator/1 -> Mux3/1, Logical Operator2/1
  Sum4/1 -> Math Function/1
  Sum2/1 -> Sum4/2
  Sum6/1 -> Relational Operator1/2
  Constant8/1 -> Sum6/2
  Deg->Rad2/1 -> Gain3/1, Sum4/1  "Beta"
  Sum3/1 -> Deg->Rad2/1
  sigma/1 -> Sum3/2
  Constant9/1 -> Sum3/1
  Relational Operator1/1 -> Logical Operator/2
  Relational Operator/1 -> Logical Operator/1
  Constant3/1 -> Relational Operator/2
  Constant1/1 -> Sum2/2

== system UnifiedPowerFlowController/UPFC Controller/SE Control (UPFC)/Firing Pulses Generator/Bridge 1Y /Phase A ==
  note: |
      | |
      | |
      | [Q1]
      | |
      | |
  note: |
      | |
      | [Q2]
      | |
      | |
  note: |
      | |
      | [Q3]
      | |
      | |
  note: |
      | |
      | [G4]
      | |
      | |
      | |
  note: --------[D_NP]---------
  note: --------[D-NN]---------
  note: ---------- A
  note: |
      | |
      | |
      | |
      | |
      | |
      | |
      | |
      | |
      | |
      | |
  note: N -------
  note: - Vdc -------------------------------
  note: + Vdc -------------------------------
  note: Q4,Q1
  note: Q2,Q3
  note: Q1,Q2,Q3,Q4
  note: |
      | |
      | |
      | |
      | |
      | |
      | |
      | |
      | |
      | |
      | |
  note: |
      | |
      | |
      | |
      | |
      | |
      | |
      | |
      | |
      | |
      | |
  note: |
      | |
      | |
      | |
      | |
      | |
      | |
      | |
      | |
      | |
      | |
  note: Pulses timing
      | ===========
  note: Normal 180deg
      | Operation
  note: Normal 180deg
      | Operation
  note: Normal 180deg
      | Operation
  note: I--------------------------------I-----------------------------I--
  note: 0
  note: 180
  note: 360
  note: ******************
  note: ******************
  note: ********************************************
  note: ******************************************
  note: Q1
  note: Q2
  note: Q3
  note: Q4
  note: |
      | |
      | |
  note: |
      | |
      | |
  note: <--Sigma-->
  wt : Inport  PortDimensions=1
  sigma : Inport  Port=2  PortDimensions=1
  D_Alpha : Inport  Port=3  PortDimensions=1
  Constant1 : Constant  Value=[0 -pi]
  Constant2 : Constant  Value=2*pi
  Constant3 : Constant  Value=0
  Constant8 : Constant  Value=pi
  Constant9 : Constant  Value=pi
  Deg->Rad2 : Gain  Gain=0.5  SaturateOnIntegerOverflow=on  OutDataTypeStr=Inherit: Same as input  ParamDataTypeStr=Inherit: Same as input
  Deg->Rad3 : Gain  Gain=-1  SaturateOnIntegerOverflow=on  OutDataTypeStr=Inherit: Same as input  ParamDataTypeStr=Inherit: Same as input
  Gain3 : Gain  Gain=2  SaturateOnIntegerOverflow=on  OutDataTypeStr=Inherit: Same as input  ParamDataTypeStr=Inherit: Same as input
  Logical Operator : Logic
  Logical Operator2 : Logic  Operator=NOT
  Math Function : Math  Operator=mod  SignedPower=on
  Mux3 : Mux  Inputs=[2 2]
  Mux4 : Mux  Inputs=2
  Relational Operator : RelationalOperator
  Relational Operator1 : RelationalOperator  Operator=<
  Selector3 : Selector  InputPortWidth=4  IndexOptions=Index vector (dialog)  Indices=[4 1 2 3]  OutputSizes=1
  Sum{2,4..6} (4 alike) : Sum  InputSameDT=on  SaturateOnIntegerOverflow=on  OutDataTypeStr=Inherit: Same as first input
  Sum3 : Sum  Inputs=+-  InputSameDT=on  SaturateOnIntegerOverflow=on  OutDataTypeStr=Inherit: Same as first input
  Pulses : Outport  VectorParamsAs1DForOutWhenUnconnected=off
  wires:
  Constant1/1 -> Sum2/2
  Constant3/1 -> Relational Operator/2
  Relational Operator/1 -> Logical Operator/1
  Relational Operator1/1 -> Logical Operator/2
  Constant9/1 -> Sum3/1
  sigma/1 -> Sum3/2
  Sum3/1 -> Deg->Rad2/1
  Deg->Rad2/1 -> Sum4/1, Gain3/1  "Beta"
  Constant8/1 -> Sum6/2
  Sum6/1 -> Relational Operator1/2
  Sum2/1 -> Sum4/2
  Sum4/1 -> Math Function/1
  Logical Operator/1 -> Logical Operator2/1, Mux3/1
  Logical Operator2/1 -> Mux3/2
  Mux3/1 -> Selector3/1
  Selector3/1 -> Pulses/1
  Gain3/1 -> Sum6/1
  Math Function/1 -> Relational Operator1/1, Relational Operator/1
  Mux4/1 -> Sum5/2
  Deg->Rad3/1 -> Mux4/2
  D_Alpha/1 -> Deg->Rad3/1, Mux4/1
  wt/1 -> Sum5/1  "wt"
  Sum5/1 -> Sum2/1  "theta"
  Constant2/1 -> Math Function/2

== system UnifiedPowerFlowController/UPFC Controller/SE Control (UPFC)/Firing Pulses Generator/Bridge 1Y /Phase B ==
  note: <--Sigma-->
  note: |
      | |
      | |
  note: |
      | |
      | |
  note: Q4
  note: Q3
  note: Q2
  note: Q1
  note: ******************************************
  note: ********************************************
  note: ******************
  note: ******************
  note: 360
  note: 180
  note: 0
  note: I--------------------------------I-----------------------------I--
  note: Normal 180deg
      | Operation
  note: Normal 180deg
      | Operation
  note: Normal 180deg
      | Operation
  note: Pulses timing
      | ===========
  note: |
      | |
      | |
      | |
      | |
      | |
      | |
      | |
      | |
      | |
      | |
  note: |
      | |
      | |
      | |
      | |
      | |
      | |
      | |
      | |
      | |
      | |
  note: |
      | |
      | |
      | |
      | |
      | |
      | |
      | |
      | |
      | |
      | |
  note: Q1,Q2,Q3,Q4
  note: Q2,Q3
  note: Q4,Q1
  note: + Vdc -------------------------------
  note: - Vdc -------------------------------
  note: N -------
  note: |
      | |
      | |
      | |
      | |
      | |
      | |
      | |
      | |
      | |
      | |
  note: ---------- A
  note: --------[D-NN]---------
  note: --------[D_NP]---------
  note: |
      | |
      | [G4]
      | |
      | |
      | |
  note: |
      | |
      | [Q3]
      | |
      | |
  note: |
      | |
      | [Q2]
      | |
      | |
  note: |
      | |
      | |
      | [Q1]
      | |
      | |
  wt : Inport  PortDimensions=1
  sigma : Inport  Port=2  PortDimensions=1
  D_Alpha : Inport  Port=3  PortDimensions=1
  Constant1 : Constant  Value=[0 -pi]
  Constant2 : Constant  Value=2*pi
  Constant3 : Constant  Value=0
  Constant8 : Constant  Value=pi
  Constant9 : Constant  Value=pi
  Deg->Rad2 : Gain  Gain=0.5  SaturateOnIntegerOverflow=on  OutDataTypeStr=Inherit: Same as input  ParamDataTypeStr=Inherit: Same as input
  Deg->Rad3 : Gain  Gain=-1  SaturateOnIntegerOverflow=on  OutDataTypeStr=Inherit: Same as input  ParamDataTypeStr=Inherit: Same as input
  Gain3 : Gain  Gain=2  SaturateOnIntegerOverflow=on  OutDataTypeStr=Inherit: Same as input  ParamDataTypeStr=Inherit: Same as input
  Logical Operator : Logic
  Logical Operator2 : Logic  Operator=NOT
  Math Function : Math  Operator=mod  SignedPower=on
  Mux3 : Mux  Inputs=[2 2]
  Mux4 : Mux  Inputs=2
  Relational Operator : RelationalOperator
  Relational Operator1 : RelationalOperator  Operator=<
  Selector3 : Selector  InputPortWidth=4  IndexOptions=Index vector (dialog)  Indices=[4 1 2 3]  OutputSizes=1
  Sum{2,4..6} (4 alike) : Sum  InputSameDT=on  SaturateOnIntegerOverflow=on  OutDataTypeStr=Inherit: Same as first input
  Sum3 : Sum  Inputs=+-  InputSameDT=on  SaturateOnIntegerOverflow=on  OutDataTypeStr=Inherit: Same as first input
  Pulses : Outport  VectorParamsAs1DForOutWhenUnconnected=off
  wires:
  Constant2/1 -> Math Function/2
  Sum5/1 -> Sum2/1  "theta"
  wt/1 -> Sum5/1  "wt"
  D_Alpha/1 -> Mux4/1, Deg->Rad3/1
  Deg->Rad3/1 -> Mux4/2
  Mux4/1 -> Sum5/2
  Math Function/1 -> Relational Operator/1, Relational Operator1/1
  Gain3/1 -> Sum6/1
  Selector3/1 -> Pulses/1
  Mux3/1 -> Selector3/1
  Logical Operator2/1 -> Mux3/2
  Logical Operator/1 -> Mux3/1, Logical Operator2/1
  Sum4/1 -> Math Function/1
  Sum2/1 -> Sum4/2
  Sum6/1 -> Relational Operator1/2
  Constant8/1 -> Sum6/2
  Deg->Rad2/1 -> Gain3/1, Sum4/1  "Beta"
  Sum3/1 -> Deg->Rad2/1
  sigma/1 -> Sum3/2
  Constant9/1 -> Sum3/1
  Relational Operator1/1 -> Logical Operator/2
  Relational Operator/1 -> Logical Operator/1
  Constant3/1 -> Relational Operator/2
  Constant1/1 -> Sum2/2

== system UnifiedPowerFlowController/UPFC Controller/SE Control (UPFC)/Firing Pulses Generator/Bridge 1Y /Phase C ==
  note: |
      | |
      | |
      | [Q1]
      | |
      | |
  note: |
      | |
      | [Q2]
      | |
      | |
  note: |
      | |
      | [Q3]
      | |
      | |
  note: |
      | |
      | [G4]
      | |
      | |
      | |
  note: --------[D_NP]---------
  note: --------[D-NN]---------
  note: ---------- A
  note: |
      | |
      | |
      | |
      | |
      | |
      | |
      | |
      | |
      | |
      | |
  note: N -------
  note: - Vdc -------------------------------
  note: + Vdc -------------------------------
  note: Q4,Q1
  note: Q2,Q3
  note: Q1,Q2,Q3,Q4
  note: |
      | |
      | |
      | |
      | |
      | |
      | |
      | |
      | |
      | |
      | |
  note: |
      | |
      | |
      | |
      | |
      | |
      | |
      | |
      | |
      | |
      | |
  note: |
      | |
      | |
      | |
      | |
      | |
      | |
      | |
      | |
      | |
      | |
  note: Pulses timing
      | ===========
  note: Normal 180deg
      | Operation
  note: Normal 180deg
      | Operation
  note: Normal 180deg
      | Operation
  note: I--------------------------------I-----------------------------I--
  note: 0
  note: 180
  note: 360
  note: ******************
  note: ******************
  note: ********************************************
  note: ******************************************
  note: Q1
  note: Q2
  note: Q3
  note: Q4
  note: |
      | |
      | |
  note: |
      | |
      | |
  note: <--Sigma-->
  wt : Inport  PortDimensions=1
  sigma : Inport  Port=2  PortDimensions=1
  D_Alpha : Inport  Port=3  PortDimensions=1
  Constant1 : Constant  Value=[0 -pi]
  Constant2 : Constant  Value=2*pi
  Constant3 : Constant  Value=0
  Constant8 : Constant  Value=pi
  Constant9 : Constant  Value=pi
  Deg->Rad2 : Gain  Gain=0.5  SaturateOnIntegerOverflow=on  OutDataTypeStr=Inherit: Same as input  ParamDataTypeStr=Inherit: Same as input
  Deg->Rad3 : Gain  Gain=-1  SaturateOnIntegerOverflow=on  OutDataTypeStr=Inherit: Same as input  ParamDataTypeStr=Inherit: Same as input
  Gain3 : Gain  Gain=2  SaturateOnIntegerOverflow=on  OutDataTypeStr=Inherit: Same as input  ParamDataTypeStr=Inherit: Same as input
  Logical Operator : Logic
  Logical Operator2 : Logic  Operator=NOT
  Math Function : Math  Operator=mod  SignedPower=on
  Mux3 : Mux  Inputs=[2 2]
  Mux4 : Mux  Inputs=2
  Relational Operator : RelationalOperator
  Relational Operator1 : RelationalOperator  Operator=<
  Selector3 : Selector  InputPortWidth=4  IndexOptions=Index vector (dialog)  Indices=[4 1 2 3]  OutputSizes=1
  Sum{2,4..6} (4 alike) : Sum  InputSameDT=on  SaturateOnIntegerOverflow=on  OutDataTypeStr=Inherit: Same as first input
  Sum3 : Sum  Inputs=+-  InputSameDT=on  SaturateOnIntegerOverflow=on  OutDataTypeStr=Inherit: Same as first input
  Pulses : Outport  VectorParamsAs1DForOutWhenUnconnected=off
  wires:
  Constant1/1 -> Sum2/2
  Constant3/1 -> Relational Operator/2
  Relational Operator/1 -> Logical Operator/1
  Relational Operator1/1 -> Logical Operator/2
  Constant9/1 -> Sum3/1
  sigma/1 -> Sum3/2
  Sum3/1 -> Deg->Rad2/1
  Deg->Rad2/1 -> Sum4/1, Gain3/1  "Beta"
  Constant8/1 -> Sum6/2
  Sum6/1 -> Relational Operator1/2
  Sum2/1 -> Sum4/2
  Sum4/1 -> Math Function/1
  Logical Operator/1 -> Logical Operator2/1, Mux3/1
  Logical Operator2/1 -> Mux3/2
  Mux3/1 -> Selector3/1
  Selector3/1 -> Pulses/1
  Gain3/1 -> Sum6/1
  Math Function/1 -> Relational Operator1/1, Relational Operator/1
  Mux4/1 -> Sum5/2
  Deg->Rad3/1 -> Mux4/2
  D_Alpha/1 -> Deg->Rad3/1, Mux4/1
  wt/1 -> Sum5/1  "wt"
  Sum5/1 -> Sum2/1  "theta"
  Constant2/1 -> Math Function/2

== system UnifiedPowerFlowController/UPFC Controller/SE Control (UPFC)/Firing Pulses Generator/Bridge 2D/Phase A ==
  note: <--Sigma-->
  note: |
      | |
      | |
  note: |
      | |
      | |
  note: Q4
  note: Q3
  note: Q2
  note: Q1
  note: ******************************************
  note: ********************************************
  note: ******************
  note: ******************
  note: 360
  note: 180
  note: 0
  note: I--------------------------------I-----------------------------I--
  note: Normal 180deg
      | Operation
  note: Normal 180deg
      | Operation
  note: Normal 180deg
      | Operation
  note: Pulses timing
      | ===========
  note: |
      | |
      | |
      | |
      | |
      | |
      | |
      | |
      | |
      | |
      | |
  note: |
      | |
      | |
      | |
      | |
      | |
      | |
      | |
      | |
      | |
      | |
  note: |
      | |
      | |
      | |
      | |
      | |
      | |
      | |
      | |
      | |
      | |
  note: Q1,Q2,Q3,Q4
  note: Q2,Q3
  note: Q4,Q1
  note: + Vdc -------------------------------
  note: - Vdc -------------------------------
  note: N -------
  note: |
      | |
      | |
      | |
      | |
      | |
      | |
      | |
      | |
      | |
      | |
  note: ---------- A
  note: --------[D-NN]---------
  note: --------[D_NP]---------
  note: |
      | |
      | [G4]
      | |
      | |
      | |
  note: |
      | |
      | [Q3]
      | |
      | |
  note: |
      | |
      | [Q2]
      | |
      | |
  note: |
      | |
      | |
      | [Q1]
      | |
      | |
  wt : Inport  PortDimensions=1
  sigma : Inport  Port=2  PortDimensions=1
  D_Alpha : Inport  Port=3  PortDimensions=1
  Constant1 : Constant  Value=[0 -pi]
  Constant2 : Constant  Value=2*pi
  Constant3 : Constant  Value=0
  Constant8 : Constant  Value=pi
  Constant9 : Constant  Value=pi
  Deg->Rad2 : Gain  Gain=0.5  SaturateOnIntegerOverflow=on  OutDataTypeStr=Inherit: Same as input  ParamDataTypeStr=Inherit: Same as input
  Deg->Rad3 : Gain  Gain=-1  SaturateOnIntegerOverflow=on  OutDataTypeStr=Inherit: Same as input  ParamDataTypeStr=Inherit: Same as input
  Gain3 : Gain  Gain=2  SaturateOnIntegerOverflow=on  OutDataTypeStr=Inherit: Same as input  ParamDataTypeStr=Inherit: Same as input
  Logical Operator : Logic
  Logical Operator2 : Logic  Operator=NOT
  Math Function : Math  Operator=mod  SignedPower=on
  Mux3 : Mux  Inputs=[2 2]
  Mux4 : Mux  Inputs=2
  Relational Operator : RelationalOperator
  Relational Operator1 : RelationalOperator  Operator=<
  Selector3 : Selector  InputPortWidth=4  IndexOptions=Index vector (dialog)  Indices=[4 1 2 3]  OutputSizes=1
  Sum{2,4..6} (4 alike) : Sum  InputSameDT=on  SaturateOnIntegerOverflow=on  OutDataTypeStr=Inherit: Same as first input
  Sum3 : Sum  Inputs=+-  InputSameDT=on  SaturateOnIntegerOverflow=on  OutDataTypeStr=Inherit: Same as first input
  Pulses : Outport  VectorParamsAs1DForOutWhenUnconnected=off
  wires:
  Constant2/1 -> Math Function/2
  Sum5/1 -> Sum2/1  "theta"
  wt/1 -> Sum5/1  "wt"
  D_Alpha/1 -> Mux4/1, Deg->Rad3/1
  Deg->Rad3/1 -> Mux4/2
  Mux4/1 -> Sum5/2
  Math Function/1 -> Relational Operator/1, Relational Operator1/1
  Gain3/1 -> Sum6/1
  Selector3/1 -> Pulses/1
  Mux3/1 -> Selector3/1
  Logical Operator2/1 -> Mux3/2
  Logical Operator/1 -> Mux3/1, Logical Operator2/1
  Sum4/1 -> Math Function/1
  Sum2/1 -> Sum4/2
  Sum6/1 -> Relational Operator1/2
  Constant8/1 -> Sum6/2
  Deg->Rad2/1 -> Gain3/1, Sum4/1  "Beta"
  Sum3/1 -> Deg->Rad2/1
  sigma/1 -> Sum3/2
  Constant9/1 -> Sum3/1
  Relational Operator1/1 -> Logical Operator/2
  Relational Operator/1 -> Logical Operator/1
  Constant3/1 -> Relational Operator/2
  Constant1/1 -> Sum2/2
